simulink model "untitled1"  (R2021a)
settings: Solver=VariableStepAuto  StartTime=0.0  StopTime=50  RelTol=1e-3
settings Model: Creator=Administrator  LastModifiedBy=Administrator

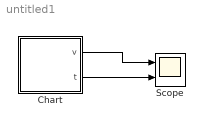
== system untitled1 ==
  Chart : Stateflow chart  TreatAsAtomicUnit=on
  Scope : Scope  NumInputPorts=2
  wires:
  Chart/1(v) -> Scope/1
  Chart/2(t) -> Scope/2

== stateflow chart untitled1/Chart ==
  state p1
    during:
    t=t+0.01;
    v=27.78-1.35*t;
  state p2
    during:
    t=t+0.01;
    v=-4.36*t+0.045*t*t+65.105;
  state p3
    during:
    t=t+0.01;
    v=0;
  (default) -> p1 : {t=0;v=27.78;}
  p1 -> p2 : [v<=5.56]
  p2 -> p3 : [v<=0]
  data: v output; t output
